simulink model "dlbsTestHarnessConcatenate4"  (R2025b)
settings: Solver=VariableStepAuto  StartTime=0.0  StopTime=10.0  RelTol=1e-3
undefined symbols (not defined in the file or in its folder): dY, X1, X2, X3, X4
libraries: dlbsBlockExtractGradientGF x4, dlbsBlockConcatenate x1, dlbsBlockInsertGradientGF x1
settings Model: Creator=lt6037  LastModifiedBy=lt6037

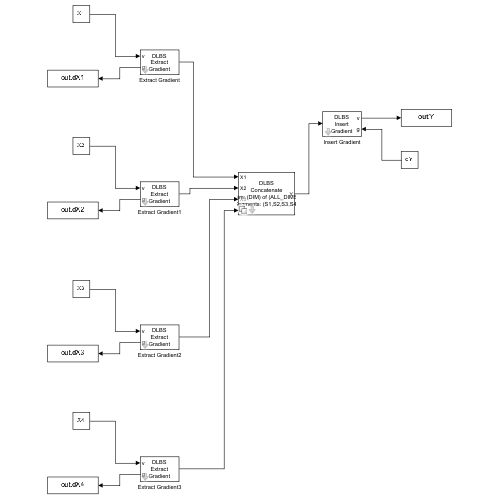
[thumbnail: Simulink's stored preview of the top-level diagram]
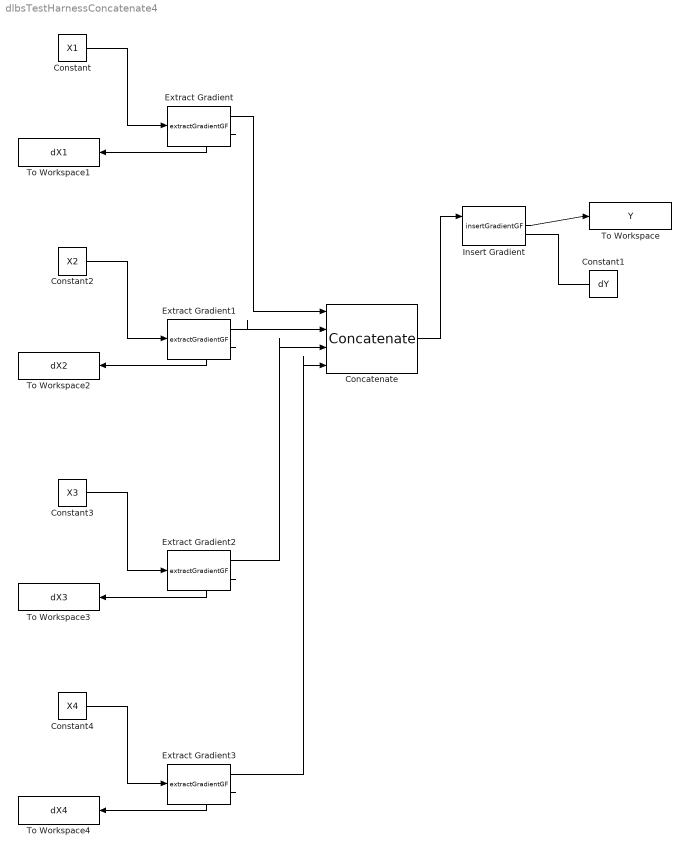
== system dlbsTestHarnessConcatenate4 ==
  Concatenate : dlbsBlockConcatenate/Concatenate  n_out=4  all_dims=ALL_DIMS  dim=DIM  s1=S1  s2=S2  s3=S3  s4=S4
  Constant : Constant  Value=X1  VectorParams1D=off
  Constant1 : Constant  Value=dY  VectorParams1D=off
  Constant2 : Constant  Value=X2  VectorParams1D=off
  Constant3 : Constant  Value=X3  VectorParams1D=off
  Constant4 : Constant  Value=X4  VectorParams1D=off
  Extract Gradient{,1..3} (4 alike) : dlbsBlockExtractGradientGF/extractGradientGF
  Insert Gradient : dlbsBlockInsertGradientGF/insertGradientGF
  To Workspace : ToWorkspace  VariableName=Y  SaveFormat=Timeseries  SampleTime=-1
      settings: MaxDataPoints=1
  To Workspace1 : ToWorkspace  VariableName=dX1  SaveFormat=Timeseries  SampleTime=-1
      settings: MaxDataPoints=1
  To Workspace2 : ToWorkspace  VariableName=dX2  SaveFormat=Timeseries  SampleTime=-1
      settings: MaxDataPoints=1
  To Workspace3 : ToWorkspace  VariableName=dX3  SaveFormat=Timeseries  SampleTime=-1
      settings: MaxDataPoints=1
  To Workspace4 : ToWorkspace  VariableName=dX4  SaveFormat=Timeseries  SampleTime=-1
      settings: MaxDataPoints=1
  wires:
  Extract Gradient/2 -> To Workspace1/1
  Constant1/1 -> Insert Gradient/2
  Insert Gradient/1 -> To Workspace/1
  Extract Gradient1/2 -> To Workspace2/1
  Constant2/1 -> Extract Gradient1/1
  Concatenate/1 -> Insert Gradient/1
  Extract Gradient/1 -> Concatenate/1
  Extract Gradient1/1 -> Concatenate/2
  Constant/1 -> Extract Gradient/1
  Extract Gradient3/1 -> Concatenate/4
  Extract Gradient3/2 -> To Workspace4/1
  Constant3/1 -> Extract Gradient2/1
  Constant4/1 -> Extract Gradient3/1
  Extract Gradient2/2 -> To Workspace3/1
  Extract Gradient2/1 -> Concatenate/3
